simulink model "GFM_L_Filter_cc"  (R2020b)
settings: Solver=ode23tb  StartTime=0.0  StopTime=Simulation_Time  FixedStep=Time_Step2  MaxStep=1e-5  RelTol=1e-3
PreLoadFcn:
  | GFM_L_Filter_Init;
InitFcn:
  | GFM_L_Filter_Init;
undefined symbols (not defined in the file): Chosen_Strategy, dur1, dur2, egfault, fb, GRD00_Lg, GRD00_Rg, Ib2, kd, Ki_cc_cp, Ki_Inertia_Less, Kp_cc_cp, kp_GFo, Kp_Inertia_Less, R, Sb, Start, Theta_Vvsc0, Time_Step, Time_Step2, Ug, Va0, Vb0, Vb1, Vb2, Vc0, Vm0, Vvsc0, wb, Zb
libraries: powerlib x25, Control_Lib x14, simulink x5, Source_Lib x1
(part 2 of 2)

== system GFM_L_Filter_cc/GFM_CC IDEAL_VSC/Control loops2/ pu P//Q computation ==
  v_abc_pu : Inport  PortDimensions=3
  i_abc_pu : Inport  Port=2  PortDimensions=3
  Demux : Demux  Outputs=3
      settings: DisplayOption=none
  Mux : Mux  Inputs=3
  Product1 : Product  InputSameDT=on  SaturateOnIntegerOverflow=on  OutDataTypeStr=Inherit: Same as first input
  Product3 : Product  InputSameDT=on  SaturateOnIntegerOverflow=on  OutDataTypeStr=Inherit: Same as first input
  Sum : Sum  Inputs=+-  InputSameDT=on  SaturateOnIntegerOverflow=on  OutDataTypeStr=Inherit: Same as first input
  Sum1 : Sum  Inputs=1  InputSameDT=on  SaturateOnIntegerOverflow=on  OutDataTypeStr=Inherit: Same as first input
  Sum4 : Sum  Inputs=1  InputSameDT=on  SaturateOnIntegerOverflow=on  OutDataTypeStr=Inherit: Same as first input
  Sum5 : Sum  Inputs=+-  InputSameDT=on  SaturateOnIntegerOverflow=on  OutDataTypeStr=Inherit: Same as first input
  Sum6 : Sum  Inputs=+-  InputSameDT=on  SaturateOnIntegerOverflow=on  OutDataTypeStr=Inherit: Same as first input
  pu->V : Gain  Gain=1/sqrt(3)  SaturateOnIntegerOverflow=on  OutDataTypeStr=Inherit: Same as input  ParamDataTypeStr=Inherit: Same as input
  pu->V1 : Gain  Gain=1/3  SaturateOnIntegerOverflow=on  OutDataTypeStr=Inherit: Same as input  ParamDataTypeStr=Inherit: Same as input
  pu->V2 : Gain  Gain=1/3  SaturateOnIntegerOverflow=on  OutDataTypeStr=Inherit: Same as input  ParamDataTypeStr=Inherit: Same as input
  P : Outport  VectorParamsAs1DForOutWhenUnconnected=off
  Q : Outport  Port=2  VectorParamsAs1DForOutWhenUnconnected=off
  wires:
  pu->V2/1 -> Q/1
  pu->V1/1 -> P/1
  Sum1/1 -> pu->V/1
  Product3/1 -> Sum1/1
  Product1/1 -> Sum4/1
  v_abc_pu/1 -> Product1/1, Demux/1
  i_abc_pu/1 -> Product1/2, Product3/2
  Sum4/1 -> pu->V1/1
  Demux/1 -> Sum/1, Sum6/2
  Demux/2 -> Sum/2, Sum5/1
  Demux/3 -> Sum5/2, Sum6/1
  Sum/1 -> Mux/3
  Sum5/1 -> Mux/1
  Sum6/1 -> Mux/2
  Mux/1 -> Product3/1
  pu->V/1 -> pu->V2/1  "Q"

== system GFM_L_Filter_cc/GFM_CC IDEAL_VSC/Control loops2/Current control ==
  Ig_dq : Inport
  Ig_dq* : Inport  Port=2
  vg_dq : Inport  Port=3
  Constant : Constant
  Current control : Subsystem
  vm : Outport  InitialOutput=0  VectorParamsAs1DForOutWhenUnconnected=off
  wires:
  Constant/1 -> Current control/4(w)
  Ig_dq/1 -> Current control/1(Is_dq)
  Ig_dq*/1 -> Current control/3(Is_dq_ref)
  vg_dq/1 -> Current control/2(Eg_dqfr)
  Current control/1(vm_dq_ref) -> vm/1

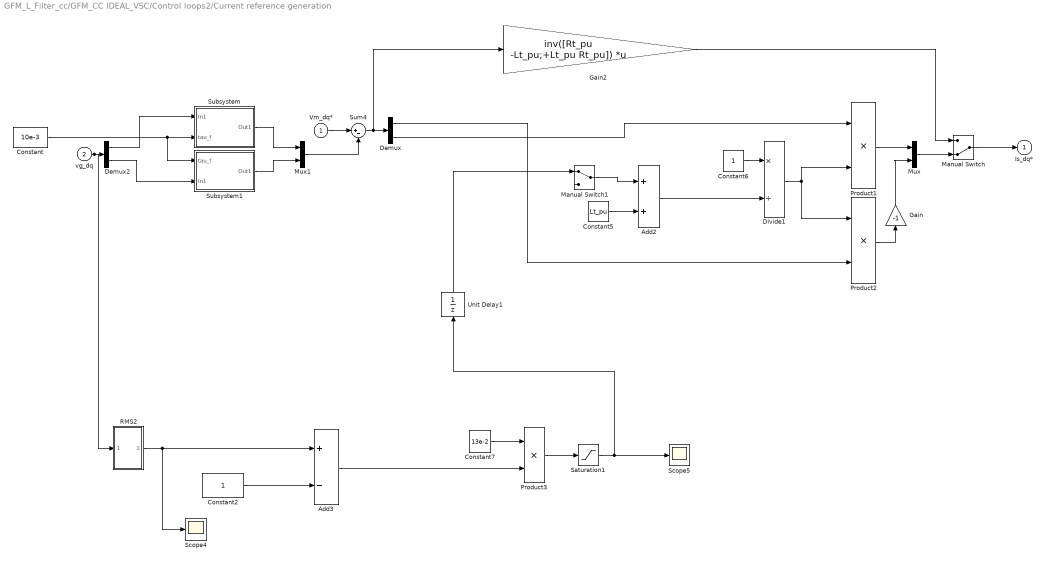
== system GFM_L_Filter_cc/GFM_CC IDEAL_VSC/Control loops2/Current reference generation ==
  Vm_dq* : Inport
  vg_dq : Inport  Port=2
  Add2 : Sum
  Add3 : Sum  Inputs=+-
  Constant : Constant  Value=10e-3
  Constant2 : Constant
  Constant5 : Constant  Value=Lt_pu
  Constant6 : Constant
  Constant7 : Constant  Value=13e-2
  Demux : Demux  Outputs=2
  Demux2 : Demux  Outputs=2
  Divide1 : Product  Inputs=*/
  Gain : Gain  Gain=-1
  Gain2 : Gain  Gain=inv([Rt_pu -Lt_pu;+Lt_pu Rt_pu])  Multiplication=Matrix(K*u)
  Manual Switch : ManualSwitch  CurrentSetting=0
  Manual Switch1 : ManualSwitch
  Mux : Mux  Inputs=2
  Mux1 : Mux  Inputs=2
  Product1 : Product
  Product2 : Product
  Product3 : Product
  RMS2 : Subsystem
  Saturation1 : Saturate  UpperLimit=0  LowerLimit=-0.14
  Scope4 : Scope
  Scope5 : Scope
  Subsystem : Subsystem
  Subsystem1 : Subsystem
  Sum4 : Sum  Inputs=|+-
  Unit Delay1 : UnitDelay  SampleTime=-1  HasFrameUpgradeWarning=on
  Is_dq* : Outport  InitialOutput=0  VectorParamsAs1DForOutWhenUnconnected=off
  wires:
  Unit Delay1/1 -> Manual Switch1/1
  Manual Switch1/1 -> Add2/1
  Vm_dq*/1 -> Sum4/1
  Demux2/2 -> Subsystem1/2(In1)
  Demux2/1 -> Subsystem/1(In1)
  Subsystem/1(Out1) -> Mux1/1
  Subsystem1/1(Out1) -> Mux1/2
  vg_dq/1 -> RMS2/1(Is_dq*), Demux2/1
  Sum4/1 -> Gain2/1, Demux/1
  Mux1/1 -> Sum4/2
  Constant/1 -> Subsystem1/1(tau_f), Subsystem/2(tau_f)
  Demux/2 -> Product1/1
  Product1/1 -> Mux/1
  Product2/1 -> Gain/1
  Demux/1 -> Product2/2
  Manual Switch/1 -> Is_dq*/1
  Gain2/1 -> Manual Switch/1
  Mux/1 -> Manual Switch/2
  Constant5/1 -> Add2/2
  Constant6/1 -> Divide1/1
  Divide1/1 -> Product2/1, Product1/2
  Gain/1 -> Mux/2
  Add2/1 -> Divide1/2
  Product3/1 -> Saturation1/1
  Constant2/1 -> Add3/2
  Constant7/1 -> Product3/1
  Add3/1 -> Product3/2
  RMS2/1(Out1) -> Add3/1, Scope4/1
  Saturation1/1 -> Unit Delay1/1, Scope5/1

== system GFM_L_Filter_cc/GFM_CC IDEAL_VSC/Control loops2/I_sat2 ==
  is_dq*+ : Inport
  Compare To Zero : simulink/Logic and Bit Operations/Compare To Zero  relop=>=  OutDataTypeStr=boolean
  Constant : Constant  Value=I_sat
  Demux : Demux  Outputs=2
  Divide : Product  Inputs=*/
  Divide1 : Product  Inputs=/*
  Mux1 : Mux  Inputs=2
  Product : Product
  Product1 : Product
  RMS : Subsystem
  Saturation1 : Saturate  UpperLimit=I_sat  LowerLimit=0
  Sum1 : Sum  Inputs=-+
  Switch : Switch  Criteria=u2 > Threshold  Threshold=0.5
  Switch1 : Switch  Criteria=u2 > Threshold  Threshold=0.5
  is_dq*sat : Outport
  sat : Outport  Port=2
  wires:
  Demux/1 -> Divide/1, Switch/3, RMS/1(d_component)
  Divide/1 -> Product/2
  Switch/1 -> Mux1/1
  Switch1/1 -> Mux1/2
  Demux/2 -> Divide1/2, Switch1/3, RMS/2(q_component)
  Divide1/1 -> Product1/2
  Product/1 -> Switch/1
  Product1/1 -> Switch1/1
  is_dq*+/1 -> Demux/1
  [sat] -> sat/1, Switch/2
  [sat] -> Switch1/2
  Compare To Zero/1 -> [sat]
  Sum1/1 -> Compare To Zero/1
  RMS/1(Module) -> Divide1/1, Sum1/2, Divide/2
  Constant/1 -> Sum1/1, Saturation1/1
  Mux1/1 -> is_dq*sat/1
  Saturation1/1 -> Product1/1, Product/1

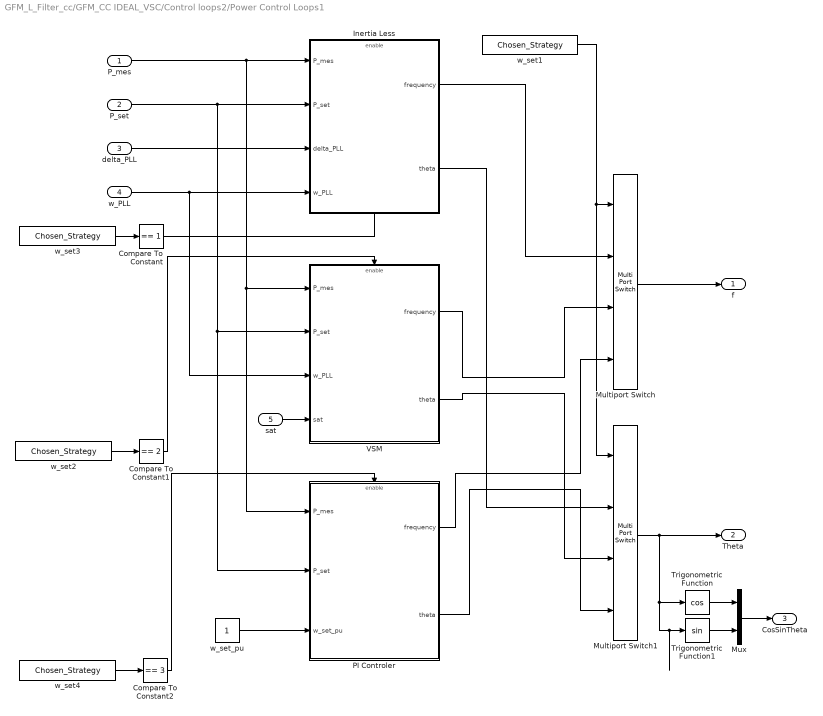
== system GFM_L_Filter_cc/GFM_CC IDEAL_VSC/Control loops2/Power Control Loops1 ==
  P_mes : Inport
  P_set : Inport  Port=2
  delta_PLL : Inport  Port=3
  w_PLL : Inport  Port=4
  sat : Inport  Port=5
  Compare To Constant : simulink/Logic and Bit Operations/Compare To Constant  relop===  const=1  OutDataTypeStr=boolean
  Compare To Constant1 : simulink/Logic and Bit Operations/Compare To Constant  relop===  const=2  OutDataTypeStr=boolean
  Compare To Constant2 : simulink/Logic and Bit Operations/Compare To Constant  relop===  const=3  OutDataTypeStr=boolean
  Inertia Less : Subsystem
  Multiport Switch : MultiPortSwitch
  Multiport Switch1 : MultiPortSwitch
  Mux : Mux  Inputs=[1 1]
  PI Controler : Subsystem
  Trigonometric Function : Trigonometry  Operator=cos
  Trigonometric Function1 : Trigonometry
  VSM : Subsystem
  w_set{1..4} (4 alike) : Constant  Value=Chosen_Strategy
  w_set_pu : Constant
  f : Outport  PortDimensions=1  VectorParamsAs1DForOutWhenUnconnected=off
  Theta : Outport  Port=2  VectorParamsAs1DForOutWhenUnconnected=off
  CosSinTheta : Outport  Port=3  PortDimensions=2  VectorParamsAs1DForOutWhenUnconnected=off
  wires:
  Trigonometric Function1/1 -> Mux/2
  Mux/1 -> CosSinTheta/1
  Trigonometric Function/1 -> Mux/1
  Compare To Constant2/1 -> PI Controler/Enable
  Compare To Constant1/1 -> VSM/Enable
  Compare To Constant/1 -> Inertia Less/Enable
  w_set4/1 -> Compare To Constant2/1
  w_set2/1 -> Compare To Constant1/1
  w_set3/1 -> Compare To Constant/1
  Inertia Less/1(frequency) -> Multiport Switch/2
  Multiport Switch/1 -> f/1
  Inertia Less/2(theta) -> Multiport Switch1/2
  VSM/2(theta) -> Multiport Switch1/3
  w_set1/1 -> Multiport Switch/1, Multiport Switch1/1
  VSM/1(frequency) -> Multiport Switch/3
  PI Controler/1(frequency) -> Multiport Switch/4
  PI Controler/2(theta) -> Multiport Switch1/4
  w_set_pu/1 -> PI Controler/3(w_set_pu)
  w_PLL/1 -> Inertia Less/4(w_PLL), VSM/3(w_PLL)
  delta_PLL/1 -> Inertia Less/3(delta_PLL)
  P_set/1 -> Inertia Less/2(P_set), PI Controler/2(P_set), VSM/2(P_set)
  P_mes/1 -> Inertia Less/1(P_mes), PI Controler/1(P_mes), VSM/1(P_mes)
  Multiport Switch1/1 -> Theta/1, Trigonometric Function1/1, Trigonometric Function/1
  sat/1 -> VSM/4(sat)

== system GFM_L_Filter_cc/GFM_CC IDEAL_VSC/Control loops2/Virtual Active Power calculation ==
  Voltage+ : Inport
  Current+ : Inport  Port=2
  Add2 : Sum
  Demux : Demux  Outputs=2
  Demux1 : Demux  Outputs=2
  Product : Product
  Product1 : Product
  Virtual Active Power : Outport
  wires:
  Product1/1 -> Add2/2
  Product/1 -> Add2/1
  Voltage+/1 -> Demux/1
  Current+/1 -> Demux1/1
  Demux/1 -> Product/2
  Demux/2 -> Product1/1
  Demux1/1 -> Product/1
  Demux1/2 -> Product1/2
  Add2/1 -> Virtual Active Power/1

== system GFM_L_Filter_cc/Generic Voltage Source/INERTIAL/CosSin ==
  Theta_rad : Inport
  Mux : Mux  Inputs=2
  Trigonometric Function : Trigonometry
  Trigonometric Function1 : Trigonometry  Operator=cos
  CosSinTheta : Outport  VectorParamsAs1DForOutWhenUnconnected=off
  wires:
  Trigonometric Function1/1 -> Mux/1
  Mux/1 -> CosSinTheta/1
  Trigonometric Function/1 -> Mux/2
  Theta_rad/1 -> Trigonometric Function1/1, Trigonometric Function/1

== system GFM_L_Filter_cc/Generic Voltage Source/INERTIAL/NetworkLeadLagTimeConstants ==
  In1 : Inport
  Constant : Constant  Value=P0
  Integrator3 : Integrator  InitialConditionSource=external  InitialCondition=(P0/Sb)*(1-TN/TD)
  Sum1 : Sum
  Sum2 : Sum  Inputs=+-
  Sum3 : Sum  Inputs=-+
  mp1 : Gain  Gain=TN/TD
  mp2 : Gain  Gain=1-TN/TD
  mp3 : Gain  Gain=1/TD
  Out1 : Outport  VectorParamsAs1DForOutWhenUnconnected=off
  wires:
  Sum3/1 -> Integrator3/2
  Integrator3/1 -> Sum2/2, Sum1/2
  Constant/1 -> Sum3/2
  Sum2/1 -> mp3/1
  mp3/1 -> Integrator3/1
  In1/1 -> mp1/1, mp2/1
  mp2/1 -> Sum2/1
  mp1/1 -> Sum1/1, Sum3/1
  Sum1/1 -> Out1/1

== system GFM_L_Filter_cc/Generic Voltage Source/INFINITE/CosSin ==
  Theta_rad : Inport
  Mux : Mux  Inputs=2
  Trigonometric Function : Trigonometry
  Trigonometric Function1 : Trigonometry  Operator=cos
  CosSinTheta : Outport  VectorParamsAs1DForOutWhenUnconnected=off
  wires:
  Trigonometric Function1/1 -> Mux/1
  Mux/1 -> CosSinTheta/1
  Trigonometric Function/1 -> Mux/2
  Theta_rad/1 -> Trigonometric Function1/1, Trigonometric Function/1

== system GFM_L_Filter_cc/Generic Voltage Source/Source_For_OP/Subsystem3 ==
  switch : Inport
  Breaker : powerlib/Elements/Breaker  InitialState=0  SwitchingTimes="[1/60  5/60]"  External=on  BreakerResistance=0.001  SnubberResistance=1e6  SnubberCapacitance=inf  Measurements=None  MoreParameters=on  NoBreakLoop=off
  Breaker1 : powerlib/Elements/Breaker  InitialState=0  SwitchingTimes="[1/60  5/60]"  External=on  BreakerResistance=0.001  SnubberResistance=1e6  SnubberCapacitance=inf  Measurements=None  MoreParameters=on  NoBreakLoop=off
  Breaker2 : powerlib/Elements/Breaker  InitialState=0  SwitchingTimes="[1/60  5/60]"  External=on  BreakerResistance=0.001  SnubberResistance=1e6  SnubberCapacitance=inf  Measurements=None  MoreParameters=on  NoBreakLoop=off
  Breaker3 : powerlib/Elements/Breaker  InitialState=1  SwitchingTimes="[1/60  5/60]"  External=on  BreakerResistance=0.001  SnubberResistance=1e6  SnubberCapacitance=inf  Measurements=None  MoreParameters=on  NoBreakLoop=off
  Breaker4 : powerlib/Elements/Breaker  InitialState=1  SwitchingTimes="[1/60  5/60]"  External=on  BreakerResistance=0.001  SnubberResistance=1e6  SnubberCapacitance=inf  Measurements=None  MoreParameters=on  NoBreakLoop=off
  Breaker5 : powerlib/Elements/Breaker  InitialState=1  SwitchingTimes="[1/60  5/60]"  External=on  BreakerResistance=0.001  SnubberResistance=1e6  SnubberCapacitance=inf  Measurements=None  MoreParameters=on  NoBreakLoop=off
  Logical Operator : Logic  Operator=NOT  AllPortsSameDT=off  OutDataTypeStr=boolean
  A : PMIOPort  Side=Left
  B : PMIOPort  Port=2  Side=Left
  C : PMIOPort  Port=3  Side=Left
  Ainit : PMIOPort  Port=4  Side=Left
  Binit : PMIOPort  Port=5  Side=Left
  Cinit : PMIOPort  Port=6  Side=Left
  a : PMIOPort  Port=7  Side=Right
  b : PMIOPort  Port=8  Side=Right
  c : PMIOPort  Port=9  Side=Right
  wires:
  switch/1 -> Breaker2/1, Breaker1/1, Breaker/1, Logical Operator/1
  Logical Operator/1 -> Breaker5/1, Breaker4/1, Breaker3/1
  connections:
  Breaker/LConn1 -- A/RConn1
  Breaker5/LConn1 -- Cinit/RConn1
  c/RConn1 -- Breaker5/RConn1 -- Breaker2/RConn1
  Breaker4/LConn1 -- Binit/RConn1
  Breaker2/LConn1 -- C/RConn1
  Breaker3/LConn1 -- Ainit/RConn1
  Breaker1/LConn1 -- B/RConn1
  Breaker/RConn1 -- Breaker3/RConn1 -- a/RConn1
  b/RConn1 -- Breaker1/RConn1 -- Breaker4/RConn1

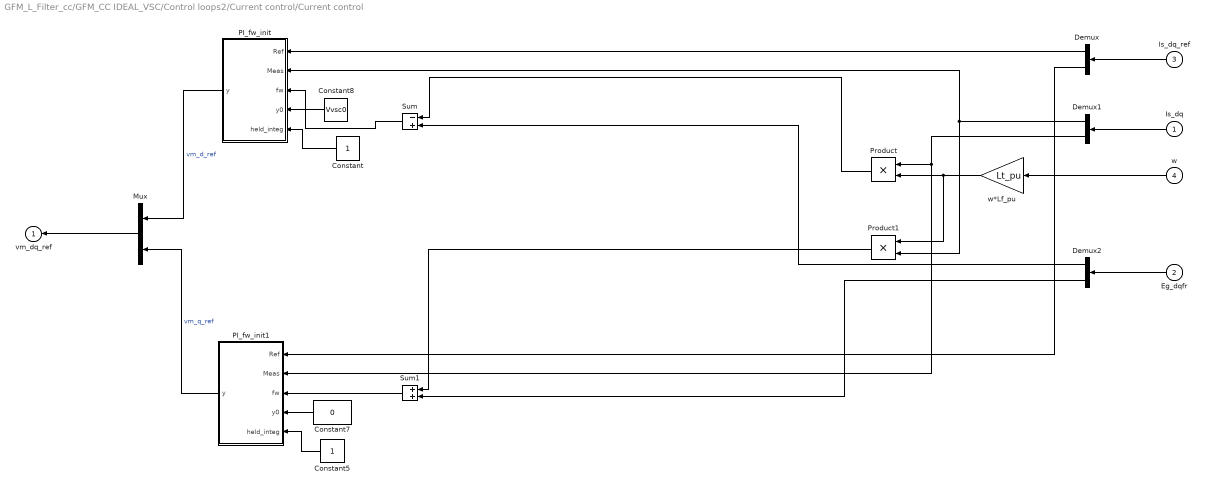
== system GFM_L_Filter_cc/GFM_CC IDEAL_VSC/Control loops2/Current control/Current control ==
  Is_dq : Inport
  Eg_dqfr : Inport  Port=2
  Is_dq_ref : Inport  Port=3
  w : Inport  Port=4
  Constant : Constant
  Constant5 : Constant
  Constant7 : Constant  Value=0
  Constant8 : Constant  Value=Vvsc0
  Demux : Demux  Outputs=2
  Demux1 : Demux  Outputs=2
  Demux2 : Demux  Outputs=2
  Mux : Mux  Inputs=[1 1]
  PI_fw_init : Subsystem  AncestorBlock=Control_Lib/PI_fw_init  TreatAsAtomicUnit=on  mask{Kp=Kp_cc_cp, Ki=Ki_cc_cp}
      mask Display:
      | color('blue')
      | text(0.3,0.5,'PI(s)')
  PI_fw_init1 : Subsystem  AncestorBlock=Control_Lib/PI_fw_init  TreatAsAtomicUnit=on  mask{Kp=Kp_cc_cp, Ki=Ki_cc_cp}
      mask Display:
      | color('blue')
      | text(0.3,0.5,'PI(s)')
  Product : Product  RndMeth=Zero
  Product1 : Product  RndMeth=Zero
  Sum : Sum  Inputs=-+
  Sum1 : Sum
  w*Lf_pu : Gain  Gain=Lt_pu
  vm_dq_ref : Outport  InitialOutput=0  VectorParamsAs1DForOutWhenUnconnected=off
  wires:
  Constant5/1 -> PI_fw_init1/5(held_integ)
  Constant/1 -> PI_fw_init/5(held_integ)
  Demux2/1 -> Sum/2
  PI_fw_init1/1(y) -> Mux/2  "vm_q_ref"
  PI_fw_init/1(y) -> Mux/1  "vm_d_ref"
  Product1/1 -> Sum1/1
  Demux/2 -> PI_fw_init1/1(Ref)
  Demux1/2 -> PI_fw_init1/2(Meas), Product/1
  w*Lf_pu/1 -> Product/2, Product1/1
  Demux1/1 -> PI_fw_init/2(Meas), Product1/2
  Demux/1 -> PI_fw_init/1(Ref)
  Is_dq_ref/1 -> Demux/1
  Is_dq/1 -> Demux1/1
  Eg_dqfr/1 -> Demux2/1
  Product/1 -> Sum/1
  Sum/1 -> PI_fw_init/3(fw)
  Sum1/1 -> PI_fw_init1/3(fw)
  w/1 -> w*Lf_pu/1
  Mux/1 -> vm_dq_ref/1
  Constant8/1 -> PI_fw_init/4(y0)
  Constant7/1 -> PI_fw_init1/4(y0)
  Demux2/2 -> Sum1/2

== system GFM_L_Filter_cc/GFM_CC IDEAL_VSC/Control loops2/Current reference generation/RMS2 ==
  Is_dq* : Inport
  Demux : Demux  Outputs=2
  Sqrt : Sqrt  SaturateOnIntegerOverflow=on
  Square : Math  Operator=square  SaturateOnIntegerOverflow=on
  Square1 : Math  Operator=square  SaturateOnIntegerOverflow=on
  Sum : Sum  Inputs=|++
  Out1 : Outport
  wires:
  Demux/2 -> Square1/1
  Is_dq*/1 -> Demux/1
  Demux/1 -> Square/1
  Sqrt/1 -> Out1/1
  Square1/1 -> Sum/2
  Square/1 -> Sum/1
  Sum/1 -> Sqrt/1

== system GFM_L_Filter_cc/GFM_CC IDEAL_VSC/Control loops2/Current reference generation/Subsystem ==
  In1 : Inport
  tau_f : Inport  Port=2
  Integrator : Integrator  InitialConditionSource=external  InitialCondition=1
  Product : Product  Inputs=/*
  Sum2 : Sum  Inputs=|+-
  Out1 : Outport
  wires:
  Product/1 -> Integrator/1
  Sum2/1 -> Product/2
  Integrator/1 -> Sum2/2, Out1/1
  tau_f/1 -> Product/1
  In1/1 -> Integrator/2, Sum2/1

== system GFM_L_Filter_cc/GFM_CC IDEAL_VSC/Control loops2/Current reference generation/Subsystem1 ==
  tau_f : Inport
  In1 : Inport  Port=2
  Integrator : Integrator  InitialConditionSource=external
  Product : Product  Inputs=/*
  Sum2 : Sum  Inputs=|+-
  Out1 : Outport
  wires:
  Product/1 -> Integrator/1
  Sum2/1 -> Product/2
  Integrator/1 -> Sum2/2, Out1/1
  In1/1 -> Sum2/1, Integrator/2
  tau_f/1 -> Product/1

== system GFM_L_Filter_cc/GFM_CC IDEAL_VSC/Control loops2/I_sat2/RMS ==
  d_component : Inport
  q_component : Inport  Port=2
  Sqrt : Sqrt  SaturateOnIntegerOverflow=on
  Square : Math  Operator=square  SaturateOnIntegerOverflow=on
  Square1 : Math  Operator=square  SaturateOnIntegerOverflow=on
  Sum : Sum  Inputs=|++
  Module : Outport
  wires:
  Sqrt/1 -> Module/1
  Square1/1 -> Sum/2
  q_component/1 -> Square1/1
  Square/1 -> Sum/1
  d_component/1 -> Square/1
  Sum/1 -> Sqrt/1

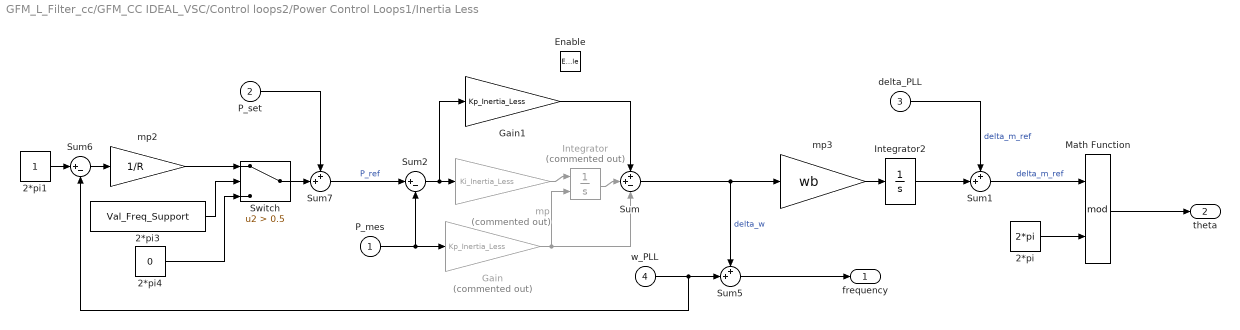
== system GFM_L_Filter_cc/GFM_CC IDEAL_VSC/Control loops2/Power Control Loops1/Inertia Less ==
  P_mes : Inport
  P_set : Inport  Port=2
  delta_PLL : Inport  Port=3
  w_PLL : Inport  Port=4
  Enable : EnablePort
  2*pi : Constant  Value=2*pi
  2*pi1 : Constant
  2*pi3 : Constant  Value=Val_Freq_Support
  2*pi4 : Constant  Value=0
  Gain : Gain  Commented=on  Gain=Kp_Inertia_Less
  Gain1 : Gain  Gain=Kp_Inertia_Less
  Integrator : Integrator  Commented=on  InitialConditionSource=external
  Integrator2 : Integrator  InitialCondition=(Theta0_VSC)*pi/180-Theta0*pi/180
  Math Function : Math  Operator=mod  SignedPower=on  SaturateOnIntegerOverflow=on
  Sum : Sum  Inputs=++-
  Sum1 : Sum  Inputs=++|
  Sum2 : Sum  Inputs=|+-
  Sum5 : Sum  Inputs=++|
  Sum6 : Sum  Inputs=|+-
  Sum7 : Sum  Inputs=++|
  Switch : Switch  Criteria=u2 > Threshold  Threshold=0.5
  mp : Gain  Commented=on  Gain=Ki_Inertia_Less
  mp2 : Gain  Gain=1/R
  mp3 : Gain  Gain=wb
  frequency : Outport  VectorParamsAs1DForOutWhenUnconnected=off
  theta : Outport  Port=2  VectorParamsAs1DForOutWhenUnconnected=off
  wires:
  Sum5/1 -> frequency/1
  Switch/1 -> Sum7/2
  Gain1/1 -> Sum/1
  Gain/1 -> Integrator/2, Sum/3
  Integrator/1 -> Sum/2
  2*pi4/1 -> Switch/3
  2*pi3/1 -> Switch/2
  mp2/1 -> Switch/1
  Integrator2/1 -> Sum1/2
  w_PLL/1 -> Sum5/2, Sum6/2
  delta_PLL/1 -> Sum1/1  "delta_m_ref"
  mp/1 -> Integrator/1
  mp3/1 -> Integrator2/1
  Sum/1 -> mp3/1, Sum5/1  "delta_w"
  Math Function/1 -> theta/1
  P_mes/1 -> Sum2/2, Gain/1
  Sum7/1 -> Sum2/1  "P_ref"
  P_set/1 -> Sum7/1
  Sum6/1 -> mp2/1
  2*pi1/1 -> Sum6/1
  2*pi/1 -> Math Function/2
  Sum1/1 -> Math Function/1  "delta_m_ref"
  Sum2/1 -> mp/1, Gain1/1

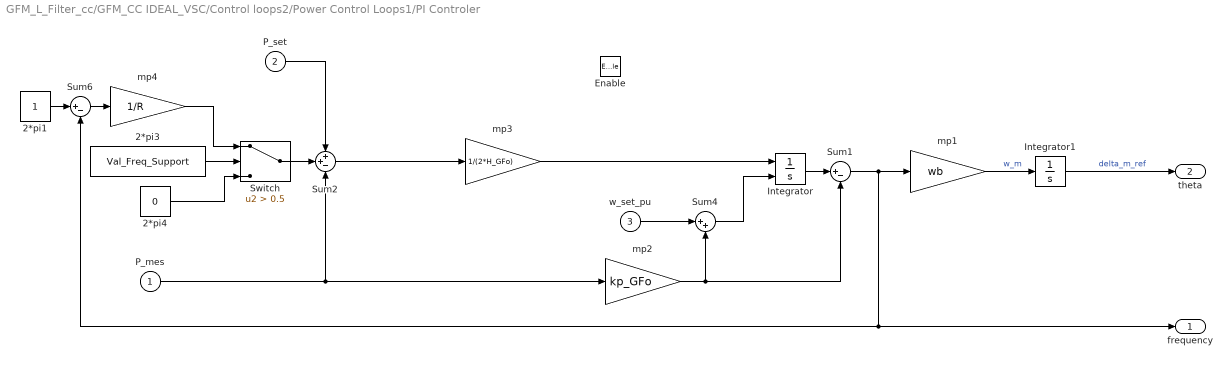
== system GFM_L_Filter_cc/GFM_CC IDEAL_VSC/Control loops2/Power Control Loops1/PI Controler ==
  P_mes : Inport
  P_set : Inport  Port=2
  w_set_pu : Inport  Port=3
  Enable : EnablePort
  2*pi1 : Constant
  2*pi3 : Constant  Value=Val_Freq_Support
  2*pi4 : Constant  Value=0
  Integrator : Integrator  InitialConditionSource=external
  Integrator1 : Integrator  InitialCondition=(Theta0_VSC)*pi/180
  Sum1 : Sum  Inputs=|+-
  Sum2 : Sum  Inputs=++-
  Sum4 : Sum  Inputs=|++
  Sum6 : Sum  Inputs=|+-
  Switch : Switch  Criteria=u2 > Threshold  Threshold=0.5
  mp1 : Gain  Gain=wb
  mp2 : Gain  Gain=kp_GFo
  mp3 : Gain  Gain=1/(2*H_GFo)
  mp4 : Gain  Gain=1/R
  frequency : Outport  VectorParamsAs1DForOutWhenUnconnected=off
  theta : Outport  Port=2  VectorParamsAs1DForOutWhenUnconnected=off
  wires:
  Switch/1 -> Sum2/2
  mp3/1 -> Integrator/1
  2*pi4/1 -> Switch/3
  Sum6/1 -> mp4/1
  2*pi3/1 -> Switch/2
  2*pi1/1 -> Sum6/1
  mp4/1 -> Switch/1
  Sum4/1 -> Integrator/2
  mp2/1 -> Sum4/2, Sum1/2
  P_mes/1 -> mp2/1, Sum2/3
  mp1/1 -> Integrator1/1  "w_m"
  Sum1/1 -> Sum6/2, frequency/1, mp1/1
  Integrator/1 -> Sum1/1
  P_set/1 -> Sum2/1
  w_set_pu/1 -> Sum4/1
  Integrator1/1 -> theta/1  "delta_m_ref"
  Sum2/1 -> mp3/1

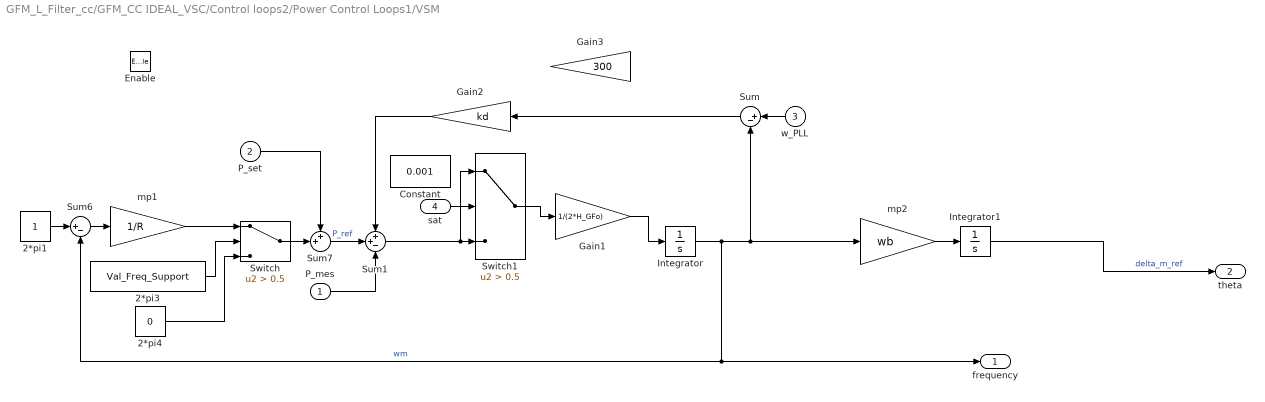
== system GFM_L_Filter_cc/GFM_CC IDEAL_VSC/Control loops2/Power Control Loops1/VSM ==
  P_mes : Inport
  P_set : Inport  Port=2
  w_PLL : Inport  Port=3
  sat : Inport  Port=4
  Enable : EnablePort
  2*pi1 : Constant
  2*pi3 : Constant  Value=Val_Freq_Support
  2*pi4 : Constant  Value=0
  Constant : Constant  Value=0.001
  Gain1 : Gain  Gain=1/(2*H_GFo)
  Gain2 : Gain  Gain=kd
  Gain3 : Gain  Gain=300
  Integrator : Integrator  InitialCondition=1
  Integrator1 : Integrator  InitialCondition=Theta0_VSC*pi/180
  Sum : Sum  Inputs=|+-
  Sum1 : Sum  Inputs=++-
  Sum6 : Sum  Inputs=|+-
  Sum7 : Sum  Inputs=++|
  Switch : Switch  Criteria=u2 > Threshold  Threshold=0.5
  Switch1 : Switch  Criteria=u2 > Threshold  Threshold=0.5
  mp1 : Gain  Gain=1/R
  mp2 : Gain  Gain=wb
  frequency : Outport  VectorParamsAs1DForOutWhenUnconnected=off
  theta : Outport  Port=2  VectorParamsAs1DForOutWhenUnconnected=off
  wires:
  Gain1/1 -> Integrator/1
  Gain2/1 -> Sum1/1
  Sum/1 -> Gain2/1
  w_PLL/1 -> Sum/1
  2*pi4/1 -> Switch/3
  2*pi3/1 -> Switch/2
  mp1/1 -> Switch/1
  2*pi1/1 -> Sum6/1
  Sum6/1 -> mp1/1
  P_set/1 -> Sum7/1
  Switch/1 -> Sum7/2
  mp2/1 -> Integrator1/1
  P_mes/1 -> Sum1/3
  Integrator/1 -> Sum6/2, frequency/1, mp2/1, Sum/2  "wm"
  Integrator1/1 -> theta/1  "delta_m_ref"
  Switch1/1 -> Gain1/1
  Sum7/1 -> Sum1/2  "P_ref"
  sat/1 -> Switch1/2
  Sum1/1 -> Switch1/1, Switch1/3

== system GFM_L_Filter_cc/GFM_CC IDEAL_VSC/Control loops2/Current control/Current control/PI_fw_init ==
  Ref : Inport
  Meas : Inport  Port=2
  fw : Inport  Port=3
  y0 : Inport  Port=4
  held_integ : Inport  Port=5
  Constant : Constant  Value=0
  Gain : Gain  Gain=Kp_cc_cp
  Gain1 : Gain  Gain=Ki_cc_cp
  Init_condition : Subsystem
  Memory : Memory  InitialCondition=1
  Subsystem : Subsystem
  Sum : Sum
  Sum1 : Sum  Inputs=+-
  Sum2 : Sum
  y : Outport  VectorParamsAs1DForOutWhenUnconnected=off
  wires:
  held_integ/1 -> Subsystem/Enable
  Subsystem/1(y) -> Sum2/2
  Init_condition/1(integ0) -> Subsystem/2(x0)
  Gain1/1 -> Subsystem/1(e)
  [comp] -> Init_condition/2(comp)
  Meas/1 -> Sum1/2
  Sum/1 -> Sum2/1, [comp]
  Sum1/1 -> Gain/1, Gain1/1
  Sum2/1 -> y/1
  y0/1 -> Init_condition/1(y0)
  Constant/1 -> Memory/1
  Memory/1 -> Init_condition/Enable
  fw/1 -> Sum/1
  Gain/1 -> Sum/2
  Ref/1 -> Sum1/1

== system GFM_L_Filter_cc/GFM_CC IDEAL_VSC/Control loops2/Current control/Current control/PI_fw_init1 ==
  Ref : Inport
  Meas : Inport  Port=2
  fw : Inport  Port=3
  y0 : Inport  Port=4
  held_integ : Inport  Port=5
  Constant : Constant  Value=0
  Gain : Gain  Gain=Kp_cc_cp
  Gain1 : Gain  Gain=Ki_cc_cp
  Init_condition : Subsystem
  Memory : Memory  InitialCondition=1
  Subsystem : Subsystem
  Sum : Sum
  Sum1 : Sum  Inputs=+-
  Sum2 : Sum
  y : Outport  VectorParamsAs1DForOutWhenUnconnected=off
  wires:
  held_integ/1 -> Subsystem/Enable
  Subsystem/1(y) -> Sum2/2
  Init_condition/1(integ0) -> Subsystem/2(x0)
  Gain1/1 -> Subsystem/1(e)
  [comp] -> Init_condition/2(comp)
  Meas/1 -> Sum1/2
  Sum/1 -> Sum2/1, [comp]
  Sum2/1 -> y/1
  y0/1 -> Init_condition/1(y0)
  Constant/1 -> Memory/1
  Memory/1 -> Init_condition/Enable
  fw/1 -> Sum/1
  Gain/1 -> Sum/2
  Sum1/1 -> Gain/1, Gain1/1
  Ref/1 -> Sum1/1

== system GFM_L_Filter_cc/GFM_CC IDEAL_VSC/Control loops2/Current control/Current control/PI_fw_init/Init_condition ==
  y0 : Inport
  comp : Inport  Port=2
  Enable : EnablePort
  Sum : Sum  Inputs=-+
  integ0 : Outport  VectorParamsAs1DForOutWhenUnconnected=off
  wires:
  Sum/1 -> integ0/1
  y0/1 -> Sum/2
  comp/1 -> Sum/1

== system GFM_L_Filter_cc/GFM_CC IDEAL_VSC/Control loops2/Current control/Current control/PI_fw_init/Subsystem ==
  e : Inport
  x0 : Inport  Port=2
  Enable : EnablePort
  Integrator : Integrator  InitialConditionSource=external
  y : Outport  VectorParamsAs1DForOutWhenUnconnected=off
  wires:
  x0/1 -> Integrator/2
  Integrator/1 -> y/1
  e/1 -> Integrator/1

== system GFM_L_Filter_cc/GFM_CC IDEAL_VSC/Control loops2/Current control/Current control/PI_fw_init1/Init_condition ==
  y0 : Inport
  comp : Inport  Port=2
  Enable : EnablePort
  Sum : Sum  Inputs=-+
  integ0 : Outport  VectorParamsAs1DForOutWhenUnconnected=off
  wires:
  Sum/1 -> integ0/1
  y0/1 -> Sum/2
  comp/1 -> Sum/1

== system GFM_L_Filter_cc/GFM_CC IDEAL_VSC/Control loops2/Current control/Current control/PI_fw_init1/Subsystem ==
  e : Inport
  x0 : Inport  Port=2
  Enable : EnablePort
  Integrator : Integrator  InitialConditionSource=external
  y : Outport  VectorParamsAs1DForOutWhenUnconnected=off
  wires:
  x0/1 -> Integrator/2
  Integrator/1 -> y/1
  e/1 -> Integrator/1
